simulink model "EX0"  (R2023b)
settings: Solver=FixedStepDiscrete  StartTime=0.0  StopTime=0.0  RelTol=1e-3
undefined symbols (not defined in the file): H, W
libraries: CPOiS_SourcesSinks x10, CPOiS_DataManipulation x3, CPOiS_Edges x1, CPOiS_General x1
settings Model: Creator=alyskawa  LastModifiedBy=alyskawa

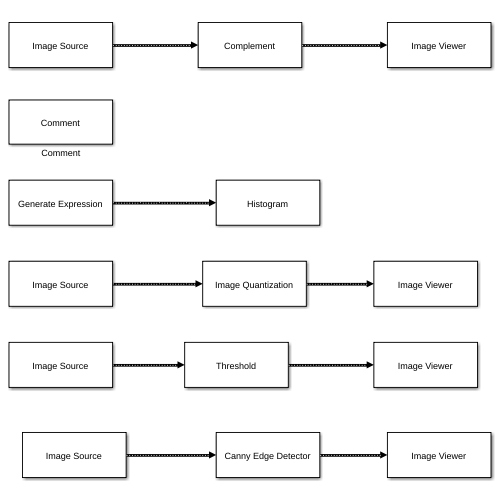
[thumbnail: Simulink's stored preview of the top-level diagram]
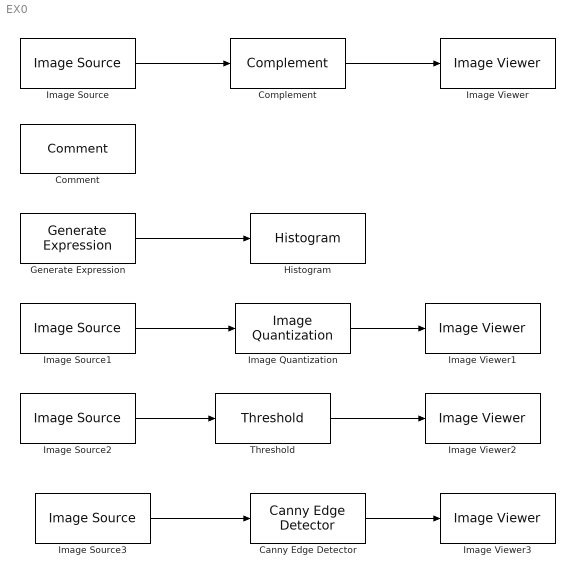
== system EX0 ==
  Canny Edge Detector : CPOiS_Edges/Canny Edge Detector  LowThresh=50  HighThresh=100
      settings: SourceProductName=CPOiS - Digital image and signal processing
  Comment : CPOiS_General/Comment
      settings: SourceProductName=CPOiS - Digital image and signal processing
  Complement : CPOiS_DataManipulation/Complement
      settings: SourceProductName=CPOiS - Digital image and signal processing
  Generate Expression : CPOiS_SourcesSinks/Generate Expression  Width=256  Height=256  Expression=W/2+H/2
      settings: SourceProductName=CPOiS - Digital image and signal processing
  Histogram : CPOiS_SourcesSinks/Histogram
      settings: SourceProductName=CPOiS - Digital image and signal processing
  Image Quantization : CPOiS_DataManipulation/Image Quantization  LevelsNum=4
      settings: SourceProductName=CPOiS - Digital image and signal processing
  Image Source{,1..3} (4 alike) : CPOiS_SourcesSinks/Image Source  FileSelection=gull.png
      settings: SourceProductName=CPOiS - Digital image and signal processing
  Image Viewer{,1..3} (4 alike) : CPOiS_SourcesSinks/Image Viewer
      settings: SourceProductName=CPOiS - Digital image and signal processing
  Threshold : CPOiS_DataManipulation/Threshold  Threshold=150
      settings: SourceProductName=CPOiS - Digital image and signal processing
  wires:
  Image Source/1 -> Complement/1
  Complement/1 -> Image Viewer/1
  Generate Expression/1 -> Histogram/1
  Image Source1/1 -> Image Quantization/1
  Image Quantization/1 -> Image Viewer1/1
  Threshold/1 -> Image Viewer2/1
  Image Source2/1 -> Threshold/1
  Image Source3/1 -> Canny Edge Detector/1
  Canny Edge Detector/1 -> Image Viewer3/1
